simulink model "iir_pipelined"  (R2024b)
settings: Solver=FixedStepDiscrete  StartTime=0.0  StopTime=10.0  FixedStep=Ts  RelTol=1e-3
PreLoadFcn:
  | if ~exist('b','var'), iir_setup; end
values from neighbouring files (symbols this model uses):
  ap = conv(a, la)    [iir_setup.m]
  bp = conv(b, la)    [iir_setup.m]
  Ts = 1/Fs    (= 2.08333333333e-05)    [iir_setup.m]
settings Model: Creator=samue  LastModifiedBy=samue
settings DataIOCC: SaveTime=off
settings DebuggingCC: ParameterPrecisionLossMsg=none

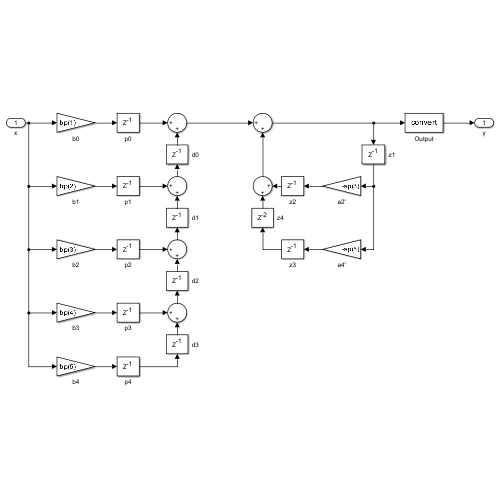
[thumbnail: Simulink's stored preview of the top-level diagram]
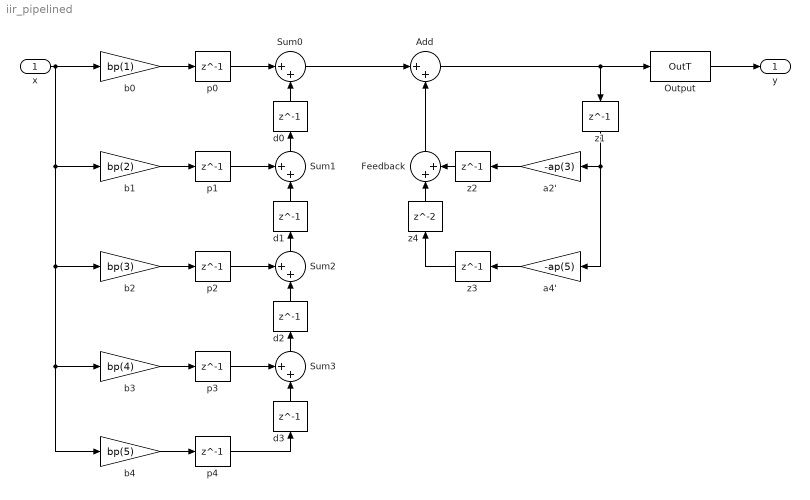
== system iir_pipelined ==
  x : Inport  OutDataTypeStr=InT  SampleTime=Ts
  Add : Sum  Inputs=|++  OutDataTypeStr=SigT
  Feedback : Sum  Inputs=|++  OutDataTypeStr=SigT
  Output : DataTypeConversion  OutDataTypeStr=OutT  RndMeth=Floor
  Sum0 : Sum  Inputs=|++  OutDataTypeStr=SigT
  Sum1 : Sum  Inputs=++|  OutDataTypeStr=SigT
  Sum2 : Sum  Inputs=++|  OutDataTypeStr=SigT
  Sum3 : Sum  Inputs=++|  OutDataTypeStr=SigT
  a2' : Gain  Gain=-ap(3)  ParamDataTypeStr=fixdt(1,CoeffWL)  OutDataTypeStr=SigT
  a4' : Gain  Gain=-ap(5)  ParamDataTypeStr=fixdt(1,CoeffWL)  OutDataTypeStr=SigT
  b0 : Gain  Gain=bp(1)  ParamDataTypeStr=fixdt(1,CoeffWL)  OutDataTypeStr=SigT
  b1 : Gain  Gain=bp(2)  ParamDataTypeStr=fixdt(1,CoeffWL)  OutDataTypeStr=SigT
  b2 : Gain  Gain=bp(3)  ParamDataTypeStr=fixdt(1,CoeffWL)  OutDataTypeStr=SigT
  b3 : Gain  Gain=bp(4)  ParamDataTypeStr=fixdt(1,CoeffWL)  OutDataTypeStr=SigT
  b4 : Gain  Gain=bp(5)  ParamDataTypeStr=fixdt(1,CoeffWL)  OutDataTypeStr=SigT
  d{0..3} (4 alike) : Delay  DelayLength=1
  p{0..4} (5 alike) : Delay  DelayLength=1
  z1 : Delay  DelayLength=1
  z2 : Delay  DelayLength=1
  z3 : Delay  DelayLength=1
  z4 : Delay
  y : Outport
  wires:
  x/1 -> b4/1, b3/1, b2/1, b1/1, b0/1
  b0/1 -> p0/1
  b1/1 -> p1/1
  b2/1 -> p2/1
  b3/1 -> p3/1
  b4/1 -> p4/1
  p0/1 -> Sum0/1
  d0/1 -> Sum0/2
  p1/1 -> Sum1/1
  d1/1 -> Sum1/2
  Sum1/1 -> d0/1
  p2/1 -> Sum2/1
  d2/1 -> Sum2/2
  Sum2/1 -> d1/1
  p3/1 -> Sum3/1
  d3/1 -> Sum3/2
  Sum3/1 -> d2/1
  p4/1 -> d3/1
  Sum0/1 -> Add/1
  Add/1 -> Output/1, z1/1
  Output/1 -> y/1
  z1/1 -> a2'/1, a4'/1
  a2'/1 -> z2/1
  z2/1 -> Feedback/2
  a4'/1 -> z3/1
  z3/1 -> z4/1
  z4/1 -> Feedback/1
  Feedback/1 -> Add/2
